simulink model "Distributor2F_Model"  (R2023a)
settings: Solver=VariableStepAuto  StartTime=0.0  StopTime=10.0  RelTol=1e-3
libraries: TimeSharedLib x4, NSA_DEVS_SINKS_ATOMIC x3, NSA_DEVS_LOGISTICS_ATOMIC x2
settings Model: Creator=david  LastModifiedBy=peter

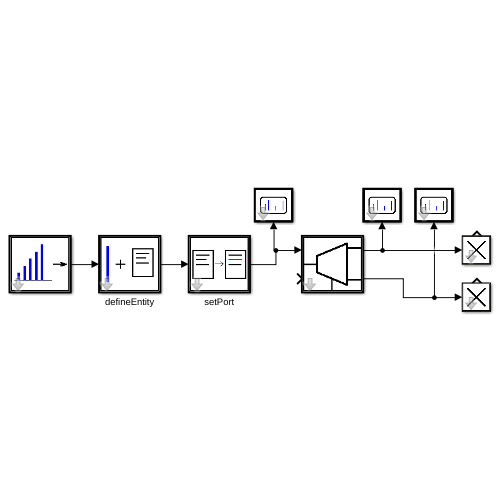
[thumbnail: Simulink's stored preview of the top-level diagram]
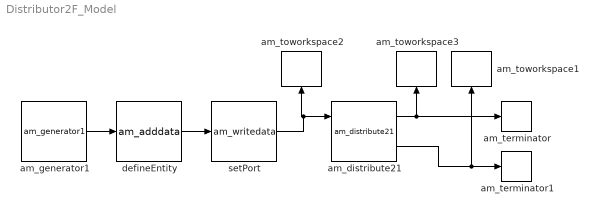
== system Distributor2F_Model ==
  am_distribute21 : TimeSharedLib/am_distribute21  port0=1  field="\"port\""  tau=[0,1]  debug=0
  am_generator1 : TimeSharedLib/am_generator1  tG=1  n0=1  nG=9  tD=[0,2]  debug=0
  am_terminator : NSA_DEVS_LOGISTICS_ATOMIC/am_terminator  tau=[0,1]  debug=0
      settings: SourceProductName=NSA_DEVS
  am_terminator1 : NSA_DEVS_LOGISTICS_ATOMIC/am_terminator  tau=[0,1]  debug=0
      settings: SourceProductName=NSA_DEVS
  am_toworkspace1 : NSA_DEVS_SINKS_ATOMIC/am_toworkspace  varname="\"dataOut2\""  t0=0  format="\"vector\""  tau=[0,3]  debug=0
      settings: SourceProductName=NSA_DEVS
  am_toworkspace2 : NSA_DEVS_SINKS_ATOMIC/am_toworkspace  varname="\"dataIn\""  t0=0  format="\"vector\""  tau=[0,3]  debug=0
      settings: SourceProductName=NSA_DEVS
  am_toworkspace3 : NSA_DEVS_SINKS_ATOMIC/am_toworkspace  varname="\"dataOut1\""  t0=0  format="\"vector\""  tau=[0,3]  debug=0
      settings: SourceProductName=NSA_DEVS
  defineEntity : TimeSharedLib/am_adddata  fields="[\"port\"]"  values="[\"1\"]"  numeric=[true]  infield="\"id\""  tau=[0,1]  debug=0
  setPort : TimeSharedLib/am_writedata  inFields=[]  outField="\"port\""  changeFunc="\"out = randi(2);\""  tau=[0,1]  debug=0
  wires:
  am_generator1/1 -> defineEntity/1
  defineEntity/1 -> setPort/1
  am_distribute21/1 -> am_terminator/1, am_toworkspace3/1
  setPort/1 -> am_distribute21/1, am_toworkspace2/1
  am_distribute21/2 -> am_terminator1/1, am_toworkspace1/1
